simulink model "SVPWM_Basic"  (R2026a)
settings: Solver=VariableStepAuto  StopTime=0.002
libraries: eePwmGeneratorTwoLevel x1

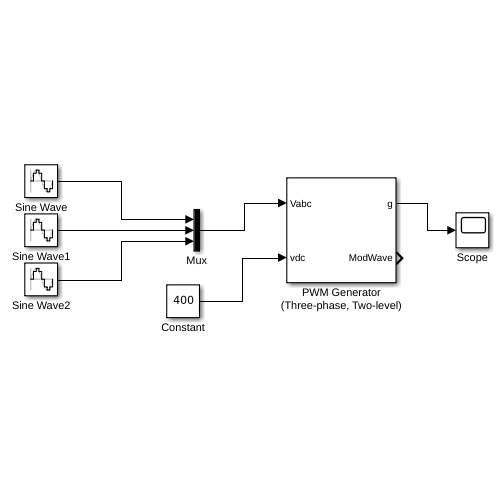
[thumbnail: Simulink's stored preview of the top-level diagram]
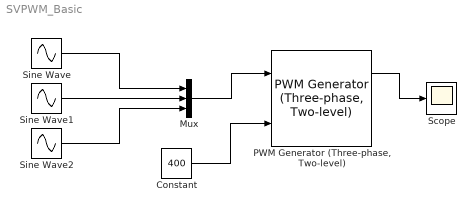
== system SVPWM_Basic ==
  Constant : Constant  Value=400
  Mux : Mux  Inputs=3
  "PWM Generator (Three-phase, Two-level)" : eePwmGeneratorTwoLevel/PWM Generator (Three-phase, Two-level)  PWMMode=Continuous PWM (CPWM)  CPWMMode=SVM: space vector modulation  DPWMMode=60 DPWM: 60 degree discontinuous PWM  fsw=5000  Ts=1e-6
      settings: LibrarySourceBlock=|
      | ee_sl_lib/Pulse Width
      | Modulation/PWM Generator
      | (Three-phase, Two-level)
  Scope : Scope
      settings: ActiveDisplayYMinimum=-0.12499999999999997  ActiveDisplayYMaximum=1.125
  Sine Wave : Sin  Amplitude=184.75  Frequency=314.159  SampleTime=1e-6
  Sine Wave1 : Sin  Amplitude=184.75  Frequency=314.159  Phase=-2.0944  SampleTime=1e-6
  Sine Wave2 : Sin  Amplitude=184.75  Frequency=314.159  Phase=+2.0944  SampleTime=1e-6
  wires:
  Sine Wave/1 -> Mux/1
  Sine Wave2/1 -> Mux/3
  Sine Wave1/1 -> Mux/2
  Mux/1 -> "PWM Generator (Three-phase, Two-level)"/1
  Constant/1 -> "PWM Generator (Three-phase, Two-level)"/2
  "PWM Generator (Three-phase, Two-level)"/1 -> Scope/1
